simulink model "OpenSeesPy_Simulink"  (R2021a)
settings: Solver=ode8  StartTime=0.0  StopTime=31.2  FixedStep=dtfast  RelTol=1e-3
PreLoadFcn:
  | initializeSimulation;
InitFcn:
  | clear('all');
  | initializeSimulation;
undefined symbols (not defined in the file): adaptive, Area, areaC, asiv, Be, Cl, coef, damperA, damperB, damperC, damperCanon, denfilter, DiscIntNeverNeededParam, dtsim, f, fir_coef, flowCanon, forceCanon, forgfact, frictionA, frictionB, frictionC, gasConstant, Gsnsr_DT, Gsnsr_FT, Kc, ke, kgap, khard, Kp, Kq, kv, learningrate, lengthCanon, massA, massB, massC, massCanon, maxDisplA, maxDisplB, maxDisplC, maxForceC, maxOilVolume, maxVelocA, maxVelocB, maxVelocC, minDisplA, minDisplB, minDisplC, minVelocA, minVelocB, minVelocC, n1siv, n2siv, Ngap, nsiv, numfilter, P_corr_i, precharge, pumpFlow ... (+25)
libraries: simulink x4, instrumentlib x2, dsparch4 x1, sldrtlib x1
(part 3 of 3)

== matlab function OpenSeesPy_Simulink/SpecimenMdl/MATLAB Function ==
  data: u input; p_r output; v_pl input; qb input; c input; v_pl output; qb output
function [p_r,v_pl,qb] = EP(u,v_pl,qb,c)
%EP nonlinear one dof element
% ElementPost = EP(u, ElementData)
%
% This is an EP material using the return mapping algorithm with kinematic
% hardening, hk.  It takes the tip displacement and returns Pr, the
% resisting force.
%
%                           [+]-->1 DOF
%                            |
%                            |
%                            |
%                            |
%                         --[+]--
%                         ///////

% Set Parameters
len        = 1;       %Element Length (in.)
k_el       = 2.9;         %Elastic Stiffness (kips/in)
Mp         = 0.2;         %Plastic Moment Capacity (kip*in)
hk         = 0.03;        %Kinematic Hardening Ratio
qb_init    = 0;           %Back force
v_pl_init  = 0;           %Element Plastic Deformation

if c == 1
    v_pl = v_pl_init;
    qb = qb_init;
end

% Get v from u
v = u/len;  %Element deformation (base rotation)

% Get q_tr (trial basic force)
q_tr = k_el * (v-v_pl);

% Determine Plastic flow parameter
n_tr   = sign(q_tr-qb);
d_beta = (n_tr*(q_tr-qb)-Mp)/(n_tr*(k_el*(1+hk))*n_tr);

if d_beta > 0
    dv_pl = n_tr*d_beta;
    q = q_tr - k_el*n_tr*d_beta;
    k = k_el * hk;
    v_pl = v_pl + dv_pl;
    qb = qb + k_el*hk*n_tr*d_beta;
else
    q = q_tr;
    k = k_el;
    v_pl = v_pl;
    qb = qb;
end

p_r = q/len;

== matlab function OpenSeesPy_Simulink/dAMB/RLS/RLS ==
  data: xm input; u input; forgfact input; dAMB_a input; P_corr_a input; dAMB output; P_corr output
function [dAMB,P_corr]  = fcn(xm,u,forgfact,dAMB_a,P_corr_a)             
        error=(u-dAMB_a'*xm);
        phik=P_corr_a*xm/(forgfact+xm'*P_corr_a*xm);
        P_corr=(P_corr_a-phik*xm'*P_corr_a)/forgfact;
        
        dAMB=dAMB_a+phik*error;
end

== matlab function OpenSeesPy_Simulink/Plant/Subsystem/Hardening-spring/MATLAB Function ==
  data: x input; Fhard output; khard input
function Fhard  = hardening(x,khard)
Fhard=khard*(x^3);

== matlab function OpenSeesPy_Simulink/Plant/Subsystem/Hysteretic/MATLAB Function ==
  data: xp input; F input; H input; Fp output; ke input; xyi input; asiv input; n1siv input; n2siv input; nsiv input; stiffdeg input; Kcur output; Fy output; strdegHmos input
function [Fp,Kcur,Fy] = stiffdegradation(xp,F,H,ke,xyi,asiv,n1siv,n2siv,nsiv,stiffdeg,strdegHmos)

Kcur=((exp(-stiffdeg*H))-asiv)*ke; 
Fyi=(1-asiv)*ke*xyi;
Fy=Fyi*(1+strdegHmos*H)^-1;
if Fy<=0.01*Fyi
    Fy=Fyi*0.01;
end
Khyst=Kcur*(1-abs(F/Fy)^(nsiv)*(n1siv*sign(F*xp)+n2siv));
Fp=Khyst*xp;

== matlab function OpenSeesPy_Simulink/Plant/Subsystem/gapclosing/MATLAB Function ==
  data: x input; Fgap output; kgap input; ke input; Ngap input; xgap input
function Fgap  = gapclosing(x,kgap,ke,Ngap,xgap)
if abs(x)<=xgap
    Fgap=0;
else
    Fgap=kgap*ke*Ngap*(abs(x)-xgap)^(Ngap-1)*x;
end
